simulink model "q_8"  (R2020a)
settings: Solver=VariableStepAuto  StartTime=0.0  StopTime=10.0  RelTol=1e-3
settings Model: EnablePacing=on  PacingRate=0.100000  Creator=INDRAJIT MARATHE  LastModifiedBy=Admin

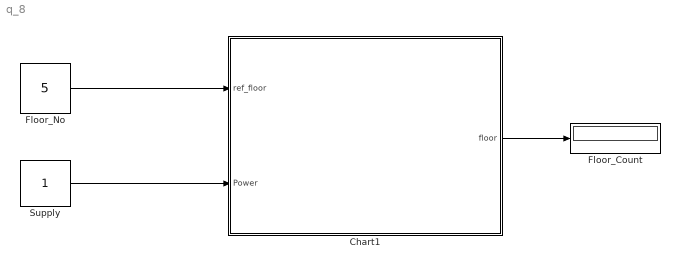
== system q_8 ==
  Chart1 : Stateflow chart  TreatAsAtomicUnit=on
      settings: PortSchema="{\"entries\":[{\"content\":{\"sides\":[{\"content\":{\"connectorIds\":[\"In2\",\"In1\"]},\"type\":\"ConnectorPlacement.EquallySpacedRectSide\",\"uuid\":\"ef9f0479-f337-4afc-9e78-8a94ba9066df\"},{\"content\":{\"connectorIds\":[\"Out1\"],\"side\":\"RIGHT\"},\"type\":\"ConnectorPlacement.EquallySpacedRectSide\",\"uuid\":\"287425df-03a5-41a8-8943-8975d18fc144\"},{\"content\":{\"connectorIds\":[],\"side\":\"TOP\"},\"type\":\"ConnectorPlacement.EquallySpacedRectSide\",\"uuid\":\"6da0e644-a717-4d0c-8dc5-4d384007fc07\"}]},\"type\":\"ConnectorPlacement.EquallySpacedConnector\",\"uuid\":\"13634f50-6146-4990-9b98-55022dda4bf9\"}],\"packageUris\":[\"http://schema.mathworks.com/mf0/Connector/19700101\"],\"version\":\"1.0\"}"
  Floor_Count : Display
  Floor_No : Constant  Value=5
  Supply : Constant
  wires:
  Floor_No/1 -> Chart1/2(ref_floor)
  Supply/1 -> Chart1/1(Power)
  Chart1/1(floor) -> Floor_Count/1

== stateflow chart q_8/Chart1 ==
  state Control [parallel]
    settings: executionOrder=1
    state Idle
      floor=0;
    state Active
    (default) -> Idle : {floor=1;}
    Idle -> Active : [Power ==1]
    Active -> Idle : [Power==0]
  state LIFT [parallel]
    settings: executionOrder=2
    state Start
    state Down
      du:floor=floor-1;
    state Up
      du:floor=floor+1;
    state Wait
    (default) -> Start
    Start -> Down [order 1] : [ref_floor<floor]
    Start -> Up [order 2] : [ref_floor>floor]
    Wait -> Start : after(5,sec)
    Down -> Wait : [floor==ref_floor]
    Up -> Wait : [floor==ref_floor]
  (default) -> Control
  data: Power input; floor output; ref_floor input
